simulink subsystem "Controlador_BA"  (R2023b)
settings: Solver=VariableStepAuto  StartTime=0.0  StopTime=10.0  RelTol=1e-3
settings Model: Creator=marqu  LastModifiedBy=marqu

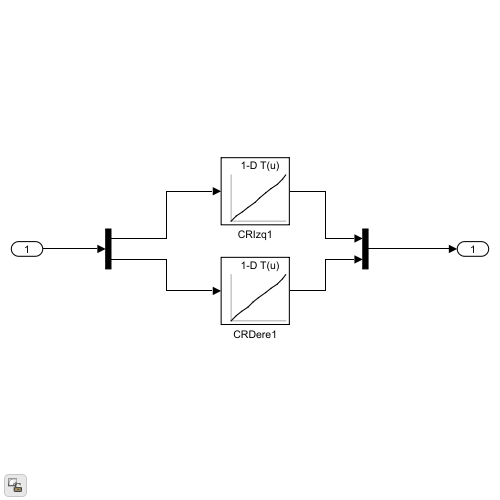
[thumbnail: Simulink's stored preview of the top-level diagram]
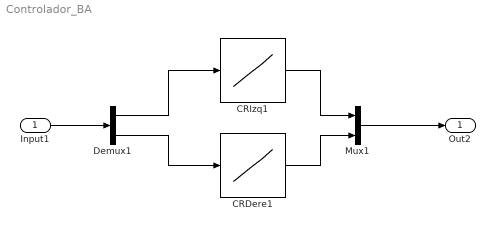
== system Controlador_BA ==
  Input1 : Inport
  CRDere1 : Lookup_n-D  NumberOfTableDimensions=1  BreakpointsForDimension1=[-0.449837893247604 -0.368067800998688 -0.272644370794296 -0.177214965224266 -0.081791520118713 0 0.122681431472301 0.218100324273109 0.313526690006256 0.395322233438492 0.449848592281342]  Table=[-255 -200 -150 -100 -50 0 50 100 150 200 255]  InternalRulePriority=Speed  RndMeth=Simplest
  CRIzq1 : Lookup_n-D  NumberOfTableDimensions=1  BreakpointsForDimension1=[-0.46346914768219 -0.368067800998688 -0.272638410329819 -0.190837785601616 -0.054527681320906 0 0.109050162136555 0.204469054937363 0.299901068210602 0.381690621376038 0.43621701002121]  Table=[-255 -200 -150 -100 -50 0 50 100 150 200 255]  InternalRulePriority=Speed  RndMeth=Simplest
  Demux1 : Demux  Outputs=2
  Mux1 : Mux  Inputs=2
  Out2 : Outport
  wires:
  CRIzq1/1 -> Mux1/1
  Demux1/2 -> CRDere1/1
  Demux1/1 -> CRIzq1/1
  CRDere1/1 -> Mux1/2
  Input1/1 -> Demux1/1
  Mux1/1 -> Out2/1
